simulink model "BpControlSystem"  (R2024b)
settings: Solver=ode45  StartTime=0.0  StopTime=1  RelTol=1e-3  EnableMultiTasking=on
libraries: neural x2
settings Model: Creator=hp  LastModifiedBy=user
settings DataIOCC: LimitDataPoints=on  SaveFormat=Array  SignalLoggingSaveFormat=ModelDataLogs  ReturnWorkspaceOutputs=off
settings OptimizationCC: InitFltsAndDblsToZero=on  LifeSpan=inf
settings DebuggingCC: SaveWithParameterizedLinksMsg=none  UnderspecifiedInitializationDetection=Classic  MergeDetectMultiDrivingBlocksExec=none  SignalResolutionControl=TryResolveAllWithWarning  MultiTaskDSMMsg=warning  MultiTaskCondExecSysMsg=none  UnconnectedInputMsg=warning  UnconnectedOutputMsg=warning  UnconnectedLineMsg=warning  SFUnexpectedBacktrackingDiag=warning  SFNoUnconditionalDefaultTransitionDiag=warning  SFExecutionAtInitializationDiag=none  ArithmeticOperatorsInVariantConditions=warning
settings HardwareCC: ProdBitPerPointer=32  ProdBitPerSizeT=32  ProdBitPerPtrDiffT=32  ProdLargestAtomicFloat=None  ProdIntDivRoundTo=Undefined  ProdEndianess=Unspecified  ProdWordSize=32  ProdHWDeviceType=32-bit Generic
settings ModelReferenceCC: EnableRefExpFcnMdlSchedulingChecks=on  PropagateSignalLabelsOutOfModel=off
settings RTWCC: GPUComputeCapability=3.5  DLArmComputeVersion=19.05
settings CodeAppCC: StateflowObjectComments=on
settings GRTTargetCC: TargetFcnLib=ansi_tfl_tmw.mat  TargetLangStandard=C89/C90 (ANSI)  CombineOutputUpdateFcns=off  GRTInterface=on
settings ConfigComp: CovMetricSettings=dw  CovSaveCumulativeToWorkspaceVar=on  CovSaveSingleToWorkspaceVar=on

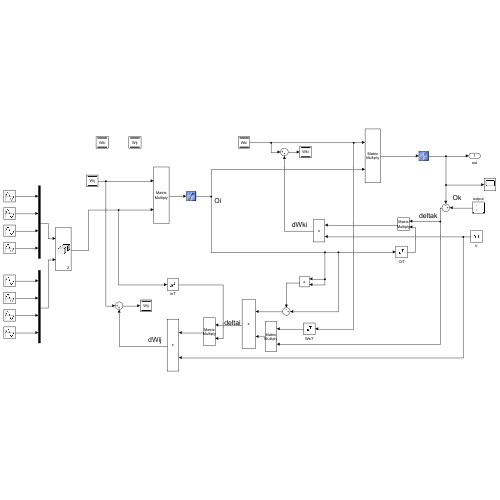
[thumbnail: Simulink's stored preview of the top-level diagram]
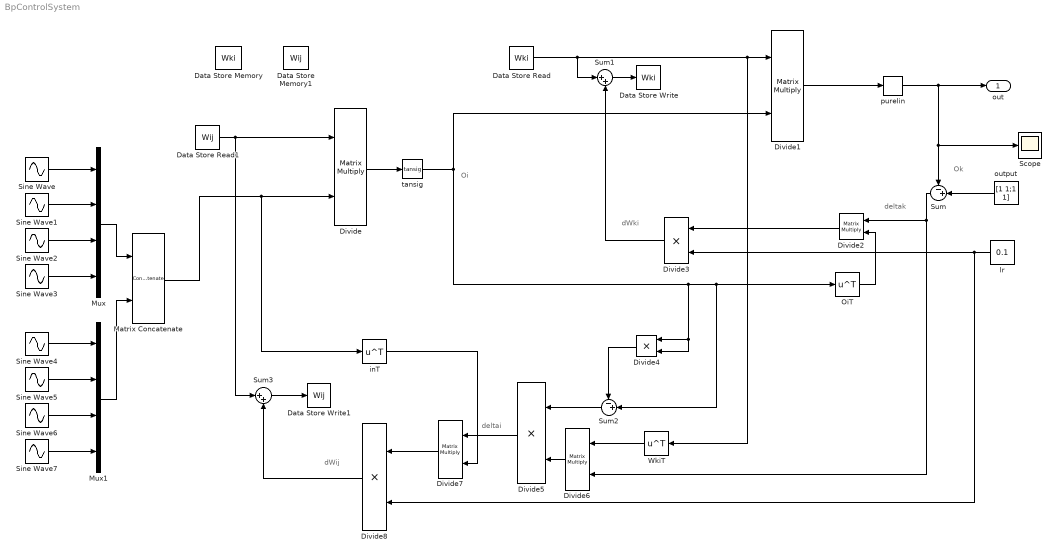
== system BpControlSystem ==
  note: deltak
  note: Oi
  note: Ok
  note: dWki
  note: dWij
  note: deltai
  Data Store Memory : DataStoreMemory  DialogController=Simulink.DDGSource  DataStoreName=Wki  InitialValue="[0.1832  -0.3349  0.7061  -0.1152  0.8087  -0.9336;0,0,0,0,0,0]"  ShowAdditionalParam=off
  Data Store Memory1 : DataStoreMemory  DialogController=Simulink.DDGSource  DataStoreName=Wij  InitialValue=|  ShowAdditionalParam=off
      | [-0.8633,  0.9231,  0.1046,  0.7128;
      |    -0.1273,  0.5248, -0.5638, -0.1951;
      |    -0.6523, -0.9853,  0.5447, -0.3640;
      |    -0.9478,  0.3601, -0.5439,  0.2173;
      |     0.9094,  0.4119, -0.2583,  0.8204;
      |    -0.1388,  0.2903,  0.7819,  0.8182]
  Data Store Read : DataStoreRead  DialogController=Simulink.DDGSource  DataStoreName=Wki  SampleTime=0  IndexOptions=Index vector (dialog)  Indices=1  OutputSizes=1
  Data Store Read1 : DataStoreRead  DialogController=Simulink.DDGSource  DataStoreName=Wij  SampleTime=0  IndexOptions=Index vector (dialog)  Indices=1  OutputSizes=1
  Data Store Write : DataStoreWrite  DialogController=Simulink.DDGSource  DataStoreName=Wki  IndexOptions=Index vector (dialog)  Indices=1  OutputSizes=1
  Data Store Write1 : DataStoreWrite  DialogController=Simulink.DDGSource  DataStoreName=Wij  IndexOptions=Index vector (dialog)  Indices=1  OutputSizes=1
  Divide : Product  Multiplication=Matrix(*)  OutDataTypeStr=Inherit: Inherit via back propagation
  Divide{1..2,6..7} (4 alike) : Product  Multiplication=Matrix(*)
  Divide{3..5,8} (4 alike) : Product
  Matrix Concatenate : Concatenate  Mode=Multidimensional array  ConcatenateDimension=2
  Mux : Mux
  Mux1 : Mux
  OiT : Math  Operator=transpose  SignedPower=on
  Scope : Scope
  Sine Wave{,1..7} (8 alike) : Sin  Amplitude=0.8  Frequency=0.0314  SampleTime=0
  Sum : Sum  Inputs=-+|
  Sum1 : Sum  Inputs=|++
  Sum2 : Sum  Inputs=-+|
  Sum3 : Sum  Inputs=|++
  WkiT : Math  Operator=transpose  SignedPower=on
  inT : Math  Operator=transpose  SignedPower=on
  lr : Constant  Value=0.1
  output : Constant  Value=[1 1;1 1]
  purelin : neural/Transfer Functions/purelin
  tansig : neural/Transfer Functions/tansig
  out : Outport
  wires:
  Divide/1 -> tansig/1
  tansig/1 -> Divide4/2, Divide4/1, OiT/1, Sum2/2, Divide1/2
  Divide1/1 -> purelin/1
  purelin/1 -> Scope/1, Sum/1, out/1
  output/1 -> Sum/2
  Sum/1 -> Divide2/1, Divide6/2
  OiT/1 -> Divide2/2
  lr/1 -> Divide3/2, Divide8/2
  Divide2/1 -> Divide3/1
  Data Store Read/1 -> Sum1/1, Divide1/1, WkiT/1
  Divide4/1 -> Sum2/1
  Sum2/1 -> Divide5/1
  WkiT/1 -> Divide6/1
  Divide6/1 -> Divide5/2
  Divide5/1 -> Divide7/1
  inT/1 -> Divide7/2
  Divide7/1 -> Divide8/1
  Divide3/1 -> Sum1/2
  Sum1/1 -> Data Store Write/1
  Data Store Read1/1 -> Divide/1, Sum3/1
  Sum3/1 -> Data Store Write1/1
  Divide8/1 -> Sum3/2
  Sine Wave/1 -> Mux/1
  Sine Wave2/1 -> Mux/3
  Sine Wave3/1 -> Mux/4
  Sine Wave6/1 -> Mux1/3
  Sine Wave4/1 -> Mux1/1
  Sine Wave5/1 -> Mux1/2
  Sine Wave7/1 -> Mux1/4
  Mux/1 -> Matrix Concatenate/1
  Sine Wave1/1 -> Mux/2
  Mux1/1 -> Matrix Concatenate/2
  Matrix Concatenate/1 -> inT/1, Divide/2
